simulink model "MSFartoystyring_2_1"  (R2018b)
settings: Solver=ode45  StartTime=tstart  StopTime=tstop  RelTol=1e-3  EnableMultiTasking=on
values from neighbouring files (symbols this model uses):
  c = 0    [find_nomoto_param.m]    (also in plotting.m; run.m)
  Delta = 900    [run.m]
  I_max = 0.15    [run.m]
  Kd = (2*damping*wn-1)/(-K)    [run.m]
  Kd_sp = -0.2    [run.m]
  Ki_LOS = 5e-6    (= 5e-06)    [run.m]
  Ki_sp = 0.001    [run.m]
  Kp = wn^2*T/-K    [run.m]
  Kp_sp = -50    [run.m]
  p0 = zeros(2,1)    [find_nomoto_param.m]    (also in plotting.m; run.m = [0,0]')
  psi0 = 0    [find_nomoto_param.m]    (also in plotting.m; run.m = 1.0471975512)
  r0 = 0    [find_nomoto_param.m]    (also in plotting.m; run.m)
  tsamp = 10    [find_nomoto_param.m]    (also in plotting.m; run.m)
  v0 = [6.63 0]'    [find_nomoto_param.m]    (also in plotting.m; run.m)
undefined symbols (not defined in the file or in its folder): msfartoystyring, WP
settings Model: ExtModeAutoUpdateStatusClock=off  Creator=christh  LastModifiedBy=dino
settings DataIOCC: LimitDataPoints=on  SaveFormat=Array  SignalLoggingSaveFormat=ModelDataLogs
settings OptimizationCC: ExpressionDepthLimit=2147483647  InitFltsAndDblsToZero=on  LifeSpan=inf
settings DebuggingCC: UnderspecifiedInitializationDetection=Classic  MergeDetectMultiDrivingBlocksExec=none  SolverPrmCheckMsg=warning  FcnCallInpInsideContextMsg=warning  StateNameClashWarn=warning  SFUnexpectedBacktrackingDiag=warning  SFNoUnconditionalDefaultTransitionDiag=warning
settings HardwareCC: ProdBitPerPointer=32  ProdBitPerSizeT=32  ProdBitPerPtrDiffT=32  ProdLargestAtomicFloat=None  ProdIntDivRoundTo=Undefined  ProdEndianess=Unspecified  ProdWordSize=32  ProdHWDeviceType=32-bit Generic
settings ModelReferenceCC: PropagateSignalLabelsOutOfModel=off
settings SFSimCC: SimUseLocalCustomCode=off
settings RTWCC: RTWUseLocalCustomCode=off
settings CodeAppCC: StateflowObjectComments=on
settings GRTTargetCC: TargetLangStandard=C89/C90 (ANSI)  GeneratePreprocessorConditionals=Disable all  CombineOutputUpdateFcns=off  GRTInterface=on
settings ConfigComp: CovMetricSettings=dw  CovHtmlReporting=on  CovSaveCumulativeToWorkspaceVar=on  CovSaveSingleToWorkspaceVar=on  CovExternalEMLEnable=off

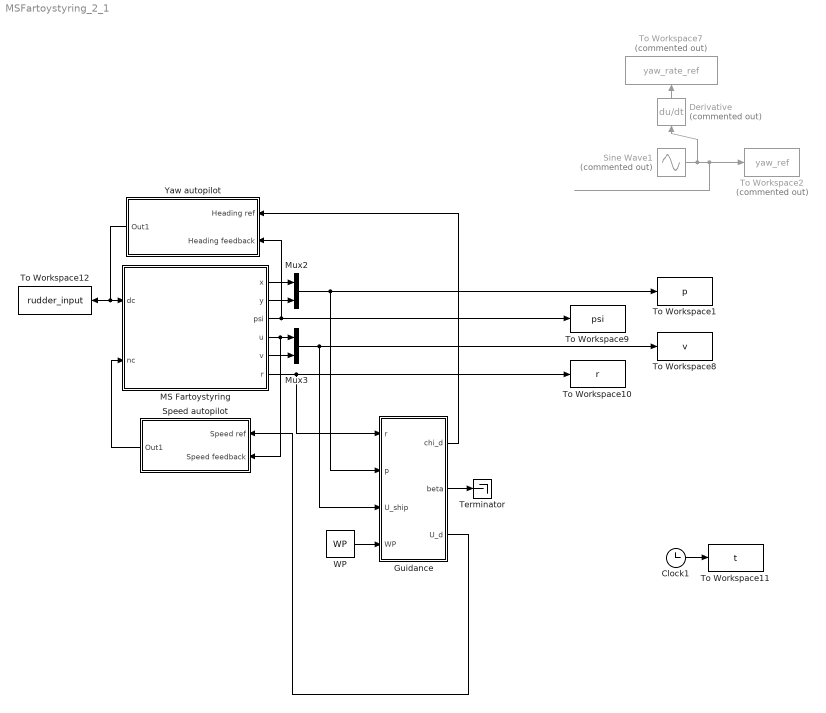
== system MSFartoystyring_2_1 ==
  Clock1 : Clock
  Derivative : Derivative  Commented=on
  Guidance : Subsystem
  MS Fartoystyring : Subsystem  mask(MS Fartoystyring for Assignment 3 G&C){x0=p0(1), y0=p0(2), u0=v0(1), v0=v0(2), psi0=psi0, r0=r0, c=c}
      mask prompts: x0 "x(t0) (m)"; y0 "y(t0) (m)"; u0 "u(t0) (m/s)"; v0 "v(t0) (m/s)"; psi0 "psi(t0) (rad)"; r0 "r(t0) (rad/s)"; c "current (0 or 1)"
      mask help:
      | Block corresponding to Figure 1 in the assignment text. Gives the response of the ship.
      |
      | The design speed of MS Fartoystyring is u=8.23 m/s.
      |
      | Input:
      | dc: commanded rudder (rad), dmax=25*pi/180
      | nc: commanded shaft speed (rad/s), nmax=85*2*pi/60
      |
      | Output:
      | x: north pos (m)
      | y: east pos (m)
      | u: surge (m/s)
      | v: sway (m/s)
      | psi: heading (rad)
      | r: yaw (rad/s)
      mask Help: Comments, bugs and help requests can be directed to the TA. Email on course website.
  Mux2 : Mux  Inputs=2
  Mux3 : Mux  Inputs=2
  Sine Wave1 : Sin  Commented=on  Amplitude=0.4  Frequency=0.004  SampleTime=0
  Speed autopilot : Subsystem
  Terminator : Terminator
  To Workspace1 : ToWorkspace  VariableName=p  SampleTime=tsamp
  To Workspace10 : ToWorkspace  VariableName=r  SampleTime=tsamp
  To Workspace11 : ToWorkspace  VariableName=t  SampleTime=tsamp
  To Workspace12 : ToWorkspace  VariableName=rudder_input  SampleTime=tsamp
  To Workspace2 : ToWorkspace  Commented=on  VariableName=yaw_ref  SampleTime=tsamp
  To Workspace7 : ToWorkspace  Commented=on  VariableName=yaw_rate_ref  SampleTime=tsamp
  To Workspace8 : ToWorkspace  VariableName=v  SampleTime=tsamp
  To Workspace9 : ToWorkspace  VariableName=psi  SampleTime=tsamp
  WP : Constant  Value=WP
  Yaw autopilot : Subsystem
  wires:
  MS Fartoystyring/5(v) -> Mux3/2
  MS Fartoystyring/6(r) -> Guidance/1(r), To Workspace10/1
  MS Fartoystyring/3(psi) -> To Workspace9/1, Yaw autopilot/2(Heading feedback)
  Clock1/1 -> To Workspace11/1
  MS Fartoystyring/1(x) -> Mux2/1
  Mux3/1 -> Guidance/3(U_ship), To Workspace8/1
  MS Fartoystyring/2(y) -> Mux2/2
  Yaw autopilot/1(Out1) -> To Workspace12/1, MS Fartoystyring/1(dc)
  MS Fartoystyring/4(u) -> Speed autopilot/2(Speed feedback), Mux3/1
  Speed autopilot/1(Out1) -> MS Fartoystyring/2(nc)
  Guidance/3(U_d) -> Speed autopilot/1(Speed ref)
  Sine Wave1/1 -> To Workspace2/1, Derivative/1
  Derivative/1 -> To Workspace7/1
  WP/1 -> Guidance/4(WP)
  Guidance/2(beta) -> Terminator/1
  Guidance/1(chi_d) -> Yaw autopilot/1(Heading ref)
  Mux2/1 -> Guidance/2(p), To Workspace1/1

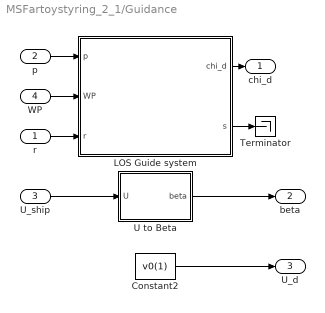
== system MSFartoystyring_2_1/Guidance ==
  r : Inport
  p : Inport  Port=2
  U_ship : Inport  Port=3
  WP : Inport  Port=4
  Constant2 : Constant  Value=v0(1)
  LOS Guide system : Subsystem  Description=LOS
  Terminator : Terminator
  U to Beta : MATLAB Function  TreatAsAtomicUnit=on
  chi_d : Outport
  beta : Outport  Port=2
  U_d : Outport  Port=3
  wires:
  U_ship/1 -> U to Beta/1(U)
  p/1 -> LOS Guide system/1(p)
  WP/1 -> LOS Guide system/2(WP)
  LOS Guide system/1(chi_d) -> chi_d/1
  U to Beta/1(beta) -> beta/1
  Constant2/1 -> U_d/1
  LOS Guide system/2(s) -> Terminator/1
  r/1 -> LOS Guide system/3(r)

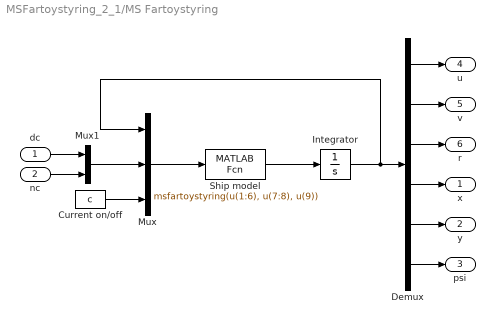
== system MSFartoystyring_2_1/MS Fartoystyring ==
  dc : Inport
  nc : Inport  Port=2
  Current on/off : Constant  Value=c
  Demux : Demux  Outputs=6
  Integrator : Integrator  InitialCondition=[u0 v0 r0 x0 y0 psi0]'
  Mux : Mux  Inputs=3
  Mux1 : Mux  Inputs=2
  Ship model : MATLABFcn  MATLABFcn=msfartoystyring(u(1:6), u(7:8), u(9))  OutputDimensions=6
  x : Outport
  y : Outport  Port=2
  psi : Outport  Port=3
  u : Outport  Port=4
  v : Outport  Port=5
  r : Outport  Port=6
  wires:
  Integrator/1 -> Mux/1, Demux/1
  Mux1/1 -> Mux/2
  dc/1 -> Mux1/1
  nc/1 -> Mux1/2
  Demux/1 -> u/1
  Demux/2 -> v/1
  Demux/3 -> r/1
  Demux/4 -> x/1
  Demux/5 -> y/1
  Demux/6 -> psi/1
  Current on/off/1 -> Mux/3
  Ship model/1 -> Integrator/1
  Mux/1 -> Ship model/1

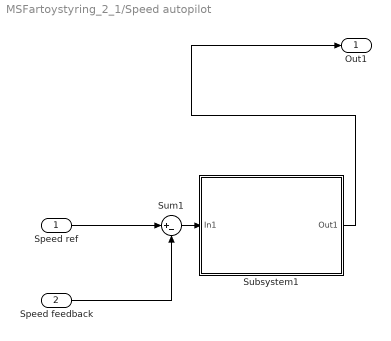
== system MSFartoystyring_2_1/Speed autopilot ==
  Speed ref : Inport
  Speed feedback : Inport  Port=2
  Subsystem1 : Subsystem
  Sum1 : Sum  Inputs=|+-
  Out1 : Outport
  wires:
  Sum1/1 -> Subsystem1/1(In1)
  Subsystem1/1(Out1) -> Out1/1
  Speed feedback/1 -> Sum1/2
  Speed ref/1 -> Sum1/1

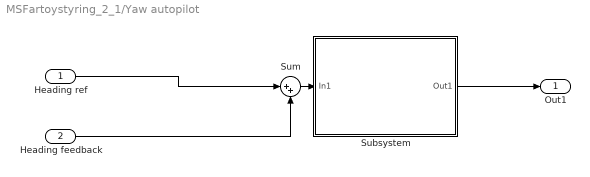
== system MSFartoystyring_2_1/Yaw autopilot ==
  Heading ref : Inport
  Heading feedback : Inport  Port=2
  Subsystem : Subsystem
  Sum : Sum  Inputs=|++
  Out1 : Outport
  wires:
  Sum/1 -> Subsystem/1(In1)
  Heading ref/1 -> Sum/1
  Subsystem/1(Out1) -> Out1/1
  Heading feedback/1 -> Sum/2

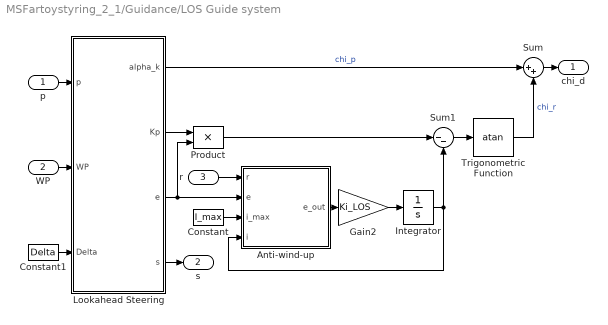
== system MSFartoystyring_2_1/Guidance/LOS Guide system ==
  p : Inport
  WP : Inport  Port=2
  r : Inport  Port=3
  Anti-wind-up : MATLAB Function  TreatAsAtomicUnit=on
  Constant : Constant  Value=I_max
  Constant1 : Constant  Value=Delta
  Gain2 : Gain  Gain=Ki_LOS
  Integrator : Integrator
  Lookahead Steering : MATLAB Function  TreatAsAtomicUnit=on
  Product : Product
  Sum : Sum  Inputs=|++
  Sum1 : Sum  Inputs=|--
  Trigonometric Function : Trigonometry  Operator=atan
  chi_d : Outport
  s : Outport  Port=2
  wires:
  WP/1 -> Lookahead Steering/2(WP)
  p/1 -> Lookahead Steering/1(p)
  Sum1/1 -> Trigonometric Function/1
  Lookahead Steering/1(alpha_k) -> Sum/1  "chi_p"
  Product/1 -> Sum1/1
  Trigonometric Function/1 -> Sum/2  "chi_r"
  Sum/1 -> chi_d/1
  Lookahead Steering/3(e) -> Anti-wind-up/2(e), Product/2
  Integrator/1 -> Sum1/2, Anti-wind-up/4(i)
  Constant/1 -> Anti-wind-up/3(i_max)
  Lookahead Steering/2(Kp) -> Product/1
  Constant1/1 -> Lookahead Steering/3(Delta)
  Lookahead Steering/4(s) -> s/1
  r/1 -> Anti-wind-up/1(r)
  Anti-wind-up/1(e_out) -> Gain2/1
  Gain2/1 -> Integrator/1

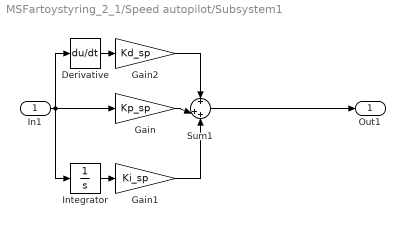
== system MSFartoystyring_2_1/Speed autopilot/Subsystem1 ==
  In1 : Inport
  Derivative : Derivative
  Gain : Gain  Gain=Kp_sp
  Gain1 : Gain  Gain=Ki_sp
  Gain2 : Gain  Gain=Kd_sp
  Integrator : Integrator
  Sum1 : Sum  Inputs=+|++
  Out1 : Outport
  wires:
  Sum1/1 -> Out1/1
  In1/1 -> Derivative/1, Integrator/1, Gain/1
  Integrator/1 -> Gain1/1
  Derivative/1 -> Gain2/1
  Gain1/1 -> Sum1/3
  Gain/1 -> Sum1/2
  Gain2/1 -> Sum1/1

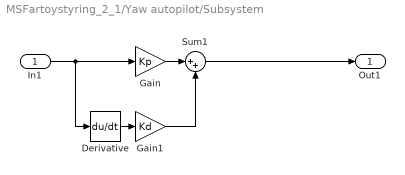
== system MSFartoystyring_2_1/Yaw autopilot/Subsystem ==
  In1 : Inport
  Derivative : Derivative
  Gain : Gain  Gain=Kp
  Gain1 : Gain  Gain=Kd
  Sum1 : Sum  Inputs=|++
  Out1 : Outport
  wires:
  Sum1/1 -> Out1/1
  Derivative/1 -> Gain1/1
  In1/1 -> Derivative/1, Gain/1
  Gain1/1 -> Sum1/2
  Gain/1 -> Sum1/1

== matlab function MSFartoystyring_2_1/Guidance/LOS Guide system/Lookahead Steering ==
  settings: updateMethod=DISCRETE  sampleTime=10
  data: p input; alpha_k output; Kp output; WP input; e output; Delta input; s output
function [alpha_k, Kp, e, s] = fcn(p, WP, Delta)
    persistent index;

    if isempty(index)
         index = 2;
    end
    % The craft's position in NED
    x = p(1);   %[m] 
    y = p(2);   %[m]    

    % The next and previous waypoint in NED
    xk = WP(1, index - 1);                  xk_1 = WP(1, index); 
    yk = WP(2, index - 1);                  yk_1 = WP(2, index);

    % How far from the desired waypoint the craft must be before going to next waypoint
    turning_Radius = 900; 

    if (((xk_1 - x)^2 + (yk_1 - y)^2) <= turning_Radius^2) && (length(WP) > index)  
        index = index + 1;
    end


    %The angle between the North and two waypoints --> atan2(dy/dx)
    alpha_k =  atan2(yk_1 - yk, xk_1 - xk); %[rad] 

    %The rotation from the NED frame to path-fixed reference frame
    Rp = [  cos(alpha_k)   -sin(alpha_k);
            sin(alpha_k)   cos(alpha_k);];

    %How far the craft is from the previous way point
    p_tilde = [x,y]' - [xk,yk]'; % or p-WP_previous

    % The coordinates of the craft in the path-fixed reference frame (Fossen p258)
    Epsilon = Rp' * p_tilde;

    % Along track distance & cross track error
    s = Epsilon(1,:);
    e = Epsilon(2,:);
    
    Kp = 1/Delta;
end

== matlab function MSFartoystyring_2_1/Guidance/U to Beta ==
  data: U input; beta output
function beta = fcn(U)
u = U(1);
v = U(2);
beta = asin(v/sqrt(u^2 +v^2));
end

== matlab function MSFartoystyring_2_1/Guidance/LOS Guide system/Anti-wind-up ==
  data: r input; e input; i_max input; e_out output; i input
function e_out = fcn(r,e,i_max, i)
if (abs(r) > 0.003) || (abs(e) > 200)
    e_out = 0;
elseif (i > i_max && e>0) || (i < -i_max && e<0)
    e_out = e/(5+4*abs(i)/i_max);
else
    e_out = e;
end
end
